simulink model "PCC_NoGearOpt_Revision"  (R2020a)
settings: Solver=ode45  StartTime=0.0  StopTime=3000  RelTol=1e-3
PreLoadFcn:
  | initial
PostLoadFcn:
  | initial
InitFcn:
  | initial
model workspace (MAT data in the model file):
  Af = Simulink.Signal
  Af.DataType = 'double'
  Af.Dimensions = -1
  Af.DimensionsMode = 'auto'
  Af.Complexity = 'real'
  Af.SampleTime = -1
  Af.SamplingMode = 'auto'
  Af.InitialValue = '4.2'
  CD = Simulink.Signal
  CD.DataType = 'double'
  CD.Dimensions = -1
  CD.DimensionsMode = 'auto'
  CD.Complexity = 'real'
  CD.SampleTime = -1
  CD.SamplingMode = 'auto'
  CD.InitialValue = '0.5'
  Delta_t = Simulink.Signal
  Delta_t.DataType = 'double'
  Delta_t.Dimensions = -1
  Delta_t.DimensionsMode = 'auto'
  Delta_t.Complexity = 'real'
  Delta_t.SampleTime = -1
  Delta_t.SamplingMode = 'auto'
  Delta_t.InitialValue = '1'
  If = Simulink.Signal
  If.DataType = 'double'
  If.Dimensions = -1
  If.DimensionsMode = 'auto'
  If.Complexity = 'real'
  If.SampleTime = -1
  If.SamplingMode = 'auto'
  If.InitialValue = '2.87'
  Ig = Simulink.Signal
  Ig.DataType = 'double'
  Ig.Dimensions = 14
  Ig.DimensionsMode = 'auto'
  Ig.Complexity = 'real'
  Ig.SampleTime = -1
  Ig.SamplingMode = 'auto'
  Ig.InitialValue = '[16.41,13.16,11.13,8.92,7.16,5.74,4.68,3.75,2.97,2.38,1.91,1.53,1.25,1]'
  L00 = Simulink.Signal
  L00.DataType = 'double'
  L00.Dimensions = -1
  L00.DimensionsMode = 'auto'
  L00.Complexity = 'real'
  L00.SampleTime = -1
  L00.SamplingMode = 'auto'
  L00.InitialValue = '-1.522'
  L01 = Simulink.Signal
  L01.DataType = 'double'
  L01.Dimensions = -1
  L01.DimensionsMode = 'auto'
  L01.Complexity = 'real'
  L01.SampleTime = -1
  L01.SamplingMode = 'auto'
  L01.InitialValue = '0.002239'
  L02 = Simulink.Signal
  L02.DataType = 'double'
  L02.Dimensions = -1
  L02.DimensionsMode = 'auto'
  L02.Complexity = 'real'
  L02.SampleTime = -1
  L02.SamplingMode = 'auto'
  L02.InitialValue = '-2.185e-07'
  L10 = Simulink.Signal
  L10.DataType = 'double'
  L10.Dimensions = -1
  L10.DimensionsMode = 'auto'
  L10.Complexity = 'real'
  L10.SampleTime = -1
  L10.SamplingMode = 'auto'
  L10.InitialValue = '0.002321'
  L11 = Simulink.Signal
  L11.DataType = 'double'
  L11.Dimensions = -1
  L11.DimensionsMode = 'auto'
  L11.Complexity = 'real'
  L11.SampleTime = -1
  L11.SamplingMode = 'auto'
  L11.InitialValue = '1.94e-06'
  L12 = Simulink.Signal
  L12.DataType = 'double'
  L12.Dimensions = -1
  L12.DimensionsMode = 'auto'
  L12.Complexity = 'real'
  L12.SampleTime = -1
  L12.SamplingMode = 'auto'
  L12.InitialValue = '4.879e-10'
  L20 = Simulink.Signal
  L20.DataType = 'double'
  L20.Dimensions = -1
  L20.DimensionsMode = 'auto'
  L20.Complexity = 'real'
  L20.SampleTime = -1
  L20.SamplingMode = 'auto'
  L20.InitialValue = '7.602e-07'
  L21 = Simulink.Signal
  L21.DataType = 'double'
  L21.Dimensions = -1
  L21.DimensionsMode = 'auto'
  L21.Complexity = 'real'
  L21.SampleTime = -1
  L21.SamplingMode = 'auto'
  L21.InitialValue = '-1.465e-09'
  L22 = Simulink.Signal
  L22.DataType = 'double'
  L22.Dimensions = -1
  L22.DimensionsMode = 'auto'
  L22.Complexity = 'real'
  L22.SampleTime = -1
  L22.SamplingMode = 'auto'
  L22.InitialValue = '9.135e-13'
  M = Simulink.Signal
  M.DataType = 'double'
  M.Dimensions = -1
  M.DimensionsMode = 'auto'
  M.Complexity = 'real'
  M.SampleTime = -1
  M.SamplingMode = 'auto'
  M.InitialValue = '49000'
  Np = Simulink.Signal
  Np.DataType = 'double'
  Np.Dimensions = -1
  Np.DimensionsMode = 'auto'
  Np.Complexity = 'real'
  Np.SampleTime = -1
  Np.SamplingMode = 'auto'
  Np.InitialValue = '50'
  Tb_min = Simulink.Signal
  Tb_min.DataType = 'double'
  Tb_min.Dimensions = -1
  Tb_min.DimensionsMode = 'auto'
  Tb_min.Complexity = 'real'
  Tb_min.SampleTime = -1
  Tb_min.SamplingMode = 'auto'
  Tb_min.InitialValue = '-20000'
  Te_max = Simulink.Signal
  Te_max.DataType = 'double'
  Te_max.Dimensions = -1
  Te_max.DimensionsMode = 'auto'
  Te_max.Complexity = 'real'
  Te_max.SampleTime = -1
  Te_max.SamplingMode = 'auto'
  Te_max.InitialValue = '2650'
  Te_min = Simulink.Signal
  Te_min.DataType = 'double'
  Te_min.Dimensions = -1
  Te_min.DimensionsMode = 'auto'
  Te_min.Complexity = 'real'
  Te_min.SampleTime = -1
  Te_min.SamplingMode = 'auto'
  Te_min.InitialValue = '-400'
  eta = Simulink.Signal
  eta.DataType = 'double'
  eta.Dimensions = -1
  eta.DimensionsMode = 'auto'
  eta.Complexity = 'real'
  eta.SampleTime = -1
  eta.SamplingMode = 'auto'
  eta.InitialValue = '0.98'
  f = Simulink.Signal
  f.DataType = 'double'
  f.Dimensions = -1
  f.DimensionsMode = 'auto'
  f.Complexity = 'real'
  f.SampleTime = -1
  f.SamplingMode = 'auto'
  f.InitialValue = '0.00743'
  g = Simulink.Signal
  g.DataType = 'double'
  g.Dimensions = -1
  g.DimensionsMode = 'auto'
  g.Complexity = 'real'
  g.SampleTime = -1
  g.SamplingMode = 'auto'
  g.InitialValue = '9.8'
  kappa_1 = Simulink.Signal
  kappa_1.DataType = 'double'
  kappa_1.Dimensions = -1
  kappa_1.DimensionsMode = 'auto'
  kappa_1.Complexity = 'real'
  kappa_1.SampleTime = -1
  kappa_1.SamplingMode = 'auto'
  kappa_1.InitialValue = '1'
  kappa_2 = Simulink.Signal
  kappa_2.DataType = 'double'
  kappa_2.Dimensions = -1
  kappa_2.DimensionsMode = 'auto'
  kappa_2.Complexity = 'real'
  kappa_2.SampleTime = -1
  kappa_2.SamplingMode = 'auto'
  kappa_2.InitialValue = '0.05'
  rho = Simulink.Signal
  rho.DataType = 'double'
  rho.Dimensions = -1
  rho.DimensionsMode = 'auto'
  rho.Complexity = 'real'
  rho.SampleTime = -1
  rho.SamplingMode = 'auto'
  rho.InitialValue = '1.225'
  rw = Simulink.Signal
  rw.DataType = 'double'
  rw.Dimensions = -1
  rw.DimensionsMode = 'auto'
  rw.Complexity = 'real'
  rw.SampleTime = -1
  rw.SamplingMode = 'auto'
  rw.InitialValue = '0.5267'
values from neighbouring files (symbols this model uses):
  EngMinTrq_Para_Value = -400    [initial.m]
  GearIni_Para_Value = 12    [initial.m]
  ParaMAP_RdSlopeOffsetAll = RdSlopeOffsetAll(5,1:2094)    [initial.m]
  ParaMAP_RdSlopeValueAll = RdSlopeValueAll(5,1:2094)    [initial.m]
  Rd_LeaderSpd = [19.4444444444 19.7511370506 20.5925623188 20.8767591057 20.2737444786 20.4902746731 20.4442142988 20.3221868298 20.2125924983 19.7727091401 19.6123069776 19.2200993307 ... (126 elements, 126x1)]    [RdLeaderSpdData.mat]
  Rd_Pos = [0:20:2500]    [LeaderSpd_Generate.m]    (also in RdLeaderSpdData.mat = [0 20 40 60 80 100 120 140 160 180 200 220 ... (126 elements)
undefined symbols (not defined in the file or in its folder): sigbuilder_block
libraries: simulink x4, Solver_SF x1
(part 1 of 2)
settings Model: SimulationMode=accelerator  Creator=LH  LastModifiedBy=luoro
settings DataIOCC: LimitDataPoints=on  SaveFormat=Array  ReturnWorkspaceOutputsName=PCC
settings OptimizationCC: BlockReduction=off  BooleanDataType=off  LifeSpan=inf
settings DebuggingCC: SaveWithParameterizedLinksMsg=none  UnderspecifiedInitializationDetection=Classic  MergeDetectMultiDrivingBlocksExec=none  SignalResolutionControl=TryResolveAllWithWarning  SFUnexpectedBacktrackingDiag=warning  SFNoUnconditionalDefaultTransitionDiag=warning  SFExecutionAtInitializationDiag=none  ArithmeticOperatorsInVariantConditions=warning
settings HardwareCC: ProdBitPerPointer=32  ProdBitPerSizeT=32  ProdBitPerPtrDiffT=32  ProdLargestAtomicFloat=None  ProdIntDivRoundTo=Undefined  ProdEndianess=Unspecified  ProdWordSize=32  ProdHWDeviceType=32-bit Generic  TargetBitPerPointer=64  TargetBitPerSizeT=64  TargetBitPerPtrDiffT=64  TargetLongLongMode=on  TargetIntDivRoundTo=Zero  TargetEndianess=LittleEndian  TargetWordSize=64  TargetHWDeviceType=MATLAB Host  ProdEqTarget=off
settings ModelReferenceCC: PropagateSignalLabelsOutOfModel=off
settings SFSimCC: SimUseLocalCustomCode=off  CustomCodeUndefinedFunction=UseInterfaceOnly
settings RTWCC: RTWUseLocalCustomCode=off
settings CodeAppCC: StateflowObjectComments=on
settings GRTTargetCC: TargetLangStandard=C89/C90 (ANSI)
settings ConfigComp: CovMetricSettings=dw  CovSaveCumulativeToWorkspaceVar=on  CovSaveSingleToWorkspaceVar=on  CovExternalEMLEnable=off  CovSFcnEnable=off

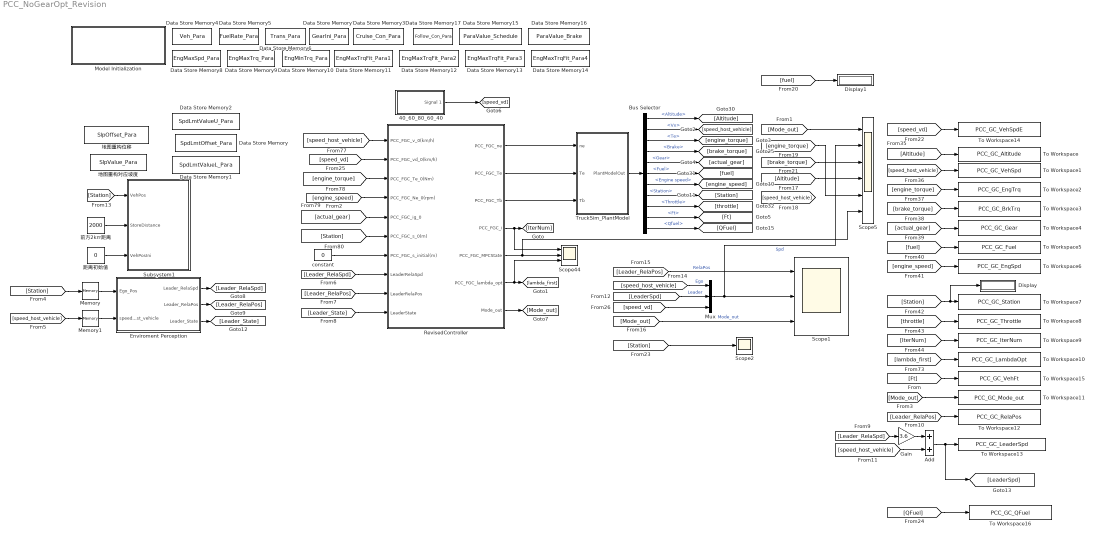
== system PCC_NoGearOpt_Revision ==
  40_60_80_60_40 : Subsystem  Tag=STV Subsys  LoadFcn=sigbuilder_block('load');  StartFcn=sigbuilder_block('start');  StopFcn=sigbuilder_block('stop');  ClipboardFcn=sigbuilder_block('clipboard');  mask(Sigbuilder block){tuvar=[0:10]}
      mask help: Simulink:masks:SigbuilderBlock_MD
      mask init:
      | if ~strcmp(get_param(bdroot(gcbh),'SimulationStatus'),'stopped') tuvar = sigbuilder_block('maskInit'); end
      settings: CopyFcn=sigbuilder_block('copy');  DeleteFcn=sigbuilder_block('delete');  ModelCloseFcn=sigbuilder_block('modelClose');  PreSaveFcn=sigbuilder_block('preSave');  PauseFcn=sigbuilder_block('pause');  ContinueFcn=sigbuilder_block('continue');  NameChangeFcn=sigbuilder_block('namechange');  OpenFcn=sigbuilder_block('open',[0 30 1440 721.5 ]);  CloseFcn=sigbuilder_block('close');
      mask Display: plot(0, 0, 100, 100,[2, 2, 32, 32, 2], [68, 8, 8, 68, 68],[32, 2], [38, 38], [32, 19, 2],[53, 60, 44], [32, 17, 17, 2],[16, 16, 31, 31]);txt = getActiveGroup(gcbh);text(2, 100, txt,'verticalAlignment', 'top');
  Add : Sum
  Bus Selector : BusSelector  OutputSignals=Altitude,Vx,Te,Brake,Gear,Fuel,Engine speed,Station,Throttle,Ft,Qfuel
  Data Store Memory : DataStoreMemory  DataStoreName=SpdLmtOffset_Para  InitialValue=ParaMAP_RdSpdLimitOffset  ShowAdditionalParam=off  OutDataTypeStr=double
  Data Store Memory1 : DataStoreMemory  DataStoreName=SpdLmtValueL_Para  InitialValue=ParaMAP_RdSpdLimitL  ShowAdditionalParam=off  OutDataTypeStr=double
  Data Store Memory10 : DataStoreMemory  DataStoreName=EngMinTrq_Para  ReadBeforeWriteMsg=warning  WriteAfterWriteMsg=warning  WriteAfterReadMsg=warning  InitialValue=EngMinTrq_Para_Value  ShowAdditionalParam=off  OutDataTypeStr=double
  Data Store Memory11 : DataStoreMemory  DataStoreName=EngMaxTrqFit_Para1  ReadBeforeWriteMsg=warning  WriteAfterWriteMsg=warning  WriteAfterReadMsg=warning  InitialValue=EngMaxTrqFit_Para_Value1  ShowAdditionalParam=off  OutDataTypeStr=double
  Data Store Memory12 : DataStoreMemory  DataStoreName=EngMaxTrqFit_Para2  ReadBeforeWriteMsg=warning  WriteAfterWriteMsg=warning  WriteAfterReadMsg=warning  InitialValue=EngMaxTrqFit_Para_Value2  ShowAdditionalParam=off  OutDataTypeStr=double
  Data Store Memory13 : DataStoreMemory  DataStoreName=EngMaxTrqFit_Para3  ReadBeforeWriteMsg=warning  WriteAfterWriteMsg=warning  WriteAfterReadMsg=warning  InitialValue=EngMaxTrqFit_Para_Value3  ShowAdditionalParam=off  OutDataTypeStr=double
  Data Store Memory14 : DataStoreMemory  DataStoreName=EngMaxTrqFit_Para4  ReadBeforeWriteMsg=warning  WriteAfterWriteMsg=warning  WriteAfterReadMsg=warning  InitialValue=EngMaxTrqFit_Para_Value4  ShowAdditionalParam=off  OutDataTypeStr=double
  Data Store Memory15 : DataStoreMemory  DataStoreName=ParaValue_Schedule  ReadBeforeWriteMsg=warning  WriteAfterWriteMsg=warning  WriteAfterReadMsg=warning  InitialValue=ParaValue_Schedule  ShowAdditionalParam=off  OutDataTypeStr=double
  Data Store Memory16 : DataStoreMemory  DataStoreName=ParaValue_Brake  ReadBeforeWriteMsg=warning  WriteAfterWriteMsg=warning  WriteAfterReadMsg=warning  InitialValue=ParaValue_Brake  ShowAdditionalParam=off  OutDataTypeStr=double
  Data Store Memory17 : DataStoreMemory  DataStoreName=Follow_Con_Para  ReadBeforeWriteMsg=warning  WriteAfterWriteMsg=warning  WriteAfterReadMsg=warning  InitialValue=Follow_Con_Para_Value  ShowAdditionalParam=off  OutDataTypeStr=double
  Data Store Memory2 : DataStoreMemory  DataStoreName=SpdLmtValueU_Para  InitialValue=ParaMAP_RdSpdLimitU  ShowAdditionalParam=off  OutDataTypeStr=double
  Data Store Memory3 : DataStoreMemory  DataStoreName=Cruise_Con_Para  ReadBeforeWriteMsg=warning  WriteAfterWriteMsg=warning  WriteAfterReadMsg=warning  InitialValue=Cruise_Con_Para_Value  ShowAdditionalParam=off  OutDataTypeStr=double
  Data Store Memory4 : DataStoreMemory  DataStoreName=Veh_Para  ReadBeforeWriteMsg=warning  WriteAfterWriteMsg=warning  WriteAfterReadMsg=warning  InitialValue=Veh_Para_Value  ShowAdditionalParam=off  OutDataTypeStr=double
  Data Store Memory5 : DataStoreMemory  DataStoreName=FuelRate_Para  ReadBeforeWriteMsg=warning  WriteAfterWriteMsg=warning  WriteAfterReadMsg=warning  InitialValue=FuelRate_Para_Value  ShowAdditionalParam=off  OutDataTypeStr=double
  Data Store Memory6 : DataStoreMemory  DataStoreName=Trans_Para  ReadBeforeWriteMsg=warning  WriteAfterWriteMsg=warning  WriteAfterReadMsg=warning  InitialValue=Trans_Para_Value  ShowAdditionalParam=off  OutDataTypeStr=double
  Data Store Memory7 : DataStoreMemory  DataStoreName=GearIni_Para  ReadBeforeWriteMsg=warning  WriteAfterWriteMsg=warning  WriteAfterReadMsg=warning  InitialValue=GearIni_Para_Value  ShowAdditionalParam=off  OutDataTypeStr=double
  Data Store Memory8 : DataStoreMemory  DataStoreName=EngMaxSpd_Para  ReadBeforeWriteMsg=warning  WriteAfterWriteMsg=warning  WriteAfterReadMsg=warning  InitialValue=EngMaxSpd_Para_Value  ShowAdditionalParam=off  OutDataTypeStr=double
  Data Store Memory9 : DataStoreMemory  DataStoreName=EngMaxTrq_Para  ReadBeforeWriteMsg=warning  WriteAfterWriteMsg=warning  WriteAfterReadMsg=warning  InitialValue=EngMaxTrq_Para_Value  ShowAdditionalParam=off  OutDataTypeStr=double
  Display : Display
      settings: Format=bank
  Display1 : Display
      settings: Format=bank
  Enviroment Perception : Subsystem
  Gain : Gain  Gain=3.6
  Memory : Memory
  Memory1 : Memory  InitialCondition=60
  Model Initialization : Subsystem  AncestorBlock=artemis/Tools /Misc/Model Initialization  mask(Model Functions){InitFcnX=initial, prel=on, posl=on, inif=on, strf=off}
      mask prompts: InitFcnX "Initialisation"; prel "Preload Function"; posl "PostLoad Function"; inif "InitFcn"; strf "StartFcn"
      mask init:
      | currentBlock = gcb;
      | root = bdroot(currentBlock);
      | 
      | if ~strcmp(get_param(root,'BlockDiagramType'),'library')
      |     if prel==1
      |         set_param(root, 'PreLoadFcn', InitFcnX);
      |     else
      |         set_param(root, 'PreLoadFcn', '');
      |     end
      |     if inif==1
      |         set_param(root, 'InitFcn', InitFcnX);
      |     else
      |         set_param(root, 'InitFcn', '');
      |     end
      |     if strf==1
      |         set_param(root, 'StartFcn', InitFcnX);
      |     else
      |         set_param(root, 'StartFcn', '');
      |     end
      |     if posl==1
      |         set_param(root, 'PostLoadFcn', InitFcnX);
      |     else
      |         set_param(root, 'PostLoadFcn', '');
      |     end
      | end
      | 
      | pos = get_param(currentBlock, 'Position');
      | width = pos(3) - pos(1); height = pos(4) - pos(2);
      | txt = [ upper(root) '\n' '- InitFcn. . . . . '  get_param(root, 'InitFcn') ];
      settings: CopyFcn=set_param(gcb,'LinkStatus','inactive')
      mask Display: text(5, height*0.5, txt, 'horizontalAlignment', 'left', 'verticalAlignment', 'middle') ;
  Mux : Mux  Inputs=3
  RevisedController : Subsystem
  Scope1 : Scope  NumInputPorts=3
  Scope2 : Scope
  Scope44 : Scope  NumInputPorts=3
  Scope5 : Scope  NumInputPorts=6
  Subsystem1 : Subsystem
  To Workspace : ToWorkspace  VariableName=PCC_GC_Altitude  SaveFormat=Structure With Time  SampleTime=0.01
      settings: Save2DSignal=2-D array (concatenate along first dimension)
  To Workspace1 : ToWorkspace  VariableName=PCC_GC_VehSpd  SaveFormat=Structure With Time  SampleTime=0.01
  To Workspace10 : ToWorkspace  VariableName=PCC_GC_LambdaOpt  SaveFormat=Structure With Time  SampleTime=0.01
  To Workspace11 : ToWorkspace  VariableName=PCC_GC_Mode_out  SaveFormat=Structure With Time  SampleTime=0.01
  To Workspace12 : ToWorkspace  VariableName=PCC_GC_RelaPos  SaveFormat=Structure With Time  SampleTime=0.01
  To Workspace13 : ToWorkspace  VariableName=PCC_GC_LeaderSpd  SaveFormat=Structure With Time  SampleTime=0.01
  To Workspace14 : ToWorkspace  VariableName=PCC_GC_VehSpdE  SaveFormat=Structure With Time  SampleTime=0.01
  To Workspace15 : ToWorkspace  VariableName=PCC_GC_VehFt  SaveFormat=Structure With Time  SampleTime=0.01
  To Workspace16 : ToWorkspace  VariableName=PCC_GC_QFuel  SaveFormat=Structure With Time  SampleTime=0.01
  To Workspace2 : ToWorkspace  VariableName=PCC_GC_EngTrq  SaveFormat=Structure With Time  SampleTime=0.01
  To Workspace3 : ToWorkspace  VariableName=PCC_GC_BrkTrq  SaveFormat=Structure With Time  SampleTime=0.01
  To Workspace4 : ToWorkspace  VariableName=PCC_GC_Gear  SaveFormat=Structure With Time  SampleTime=0.01
  To Workspace5 : ToWorkspace  VariableName=PCC_GC_Fuel  SaveFormat=Structure With Time  SampleTime=0.01
  To Workspace6 : ToWorkspace  VariableName=PCC_GC_EngSpd  SaveFormat=Structure With Time  SampleTime=0.01
  To Workspace7 : ToWorkspace  VariableName=PCC_GC_Station  SaveFormat=Structure With Time  SampleTime=0.01
  To Workspace8 : ToWorkspace  VariableName=PCC_GC_Throttle  SaveFormat=Structure With Time  SampleTime=0.01
  To Workspace9 : ToWorkspace  VariableName=PCC_GC_IterNum  SaveFormat=Structure With Time  SampleTime=0.01
  TruckSim_PlantModel : Subsystem
  constant : Constant  Value=0
  前方2km距离 : Constant  Value=2000
  地图重构位移 : DataStoreMemory  DataStoreName=SlpOffset_Para  InitialValue=ParaMAP_RdSlopeOffsetFirst200  ShowAdditionalParam=off  OutDataTypeStr=double
  地图重构对应坡度 : DataStoreMemory  DataStoreName=SlpValue_Para  InitialValue=ParaMAP_RdSlopeValueFirst200  ShowAdditionalParam=off  OutDataTypeStr=double
  距离初始值 : Constant  Value=0
  wires:
  [Altitude] -> Scope5/4
  [engine_torque] -> Scope5/5
  [fuel] -> Display1/1
  [Altitude] -> To Workspace/1
  [speed_host_vehicle] -> To Workspace1/1
  [engine_torque] -> To Workspace2/1
  [brake_torque] -> To Workspace3/1
  [actual_gear] -> To Workspace4/1
  [fuel] -> To Workspace5/1
  [engine_speed] -> To Workspace6/1
  [Station] -> Display/1, To Workspace7/1
  [throttle] -> To Workspace8/1
  [IterNum] -> To Workspace9/1
  [Station] -> Subsystem1/1(VehPos)
  前方2km距离/1 -> Subsystem1/2(StoreDistance)
  距离初始值/1 -> Subsystem1/3(VehPosIni)
  [lambda_first] -> To Workspace10/1
  RevisedController/1(PCC_FGC_ne) -> TruckSim_PlantModel/1(ne)
  RevisedController/2(PCC_FGC_Te) -> TruckSim_PlantModel/2(Te)
  [speed_host_vehicle] -> RevisedController/1(PCC_FGC_v_0(km/h))
  [engine_torque] -> RevisedController/3(PCC_FGC_Te_0(Nm))
  [actual_gear] -> RevisedController/5(PCC_FGC_ig_0)
  [Station] -> RevisedController/6(PCC_FGC_s_0(m))
  constant/1 -> RevisedController/7(PCC_FGC_s_initial(m))
  TruckSim_PlantModel/1(PlantModelOut) -> Bus Selector/1
  Bus Selector/2 -> [speed_host_vehicle]  "<Vx>"
  Bus Selector/1 -> [Altitude]  "<Altitude>"
  Bus Selector/3 -> [engine_torque]  "<Te>"
  Bus Selector/4 -> [brake_torque]  "<Brake>"
  Bus Selector/5 -> [actual_gear]  "<Gear>"
  Bus Selector/6 -> [fuel]  "<Fuel>"
  Bus Selector/7 -> [engine_speed]  "<Engine speed>"
  Bus Selector/8 -> [Station]  "<Station>"
  Bus Selector/9 -> [throttle]  "<Throttle>"
  Bus Selector/10 -> [Ft]  "<Ft>"
  [Ft] -> To Workspace15/1
  [Mode_out] -> Scope5/1
  RevisedController/4(PCC_FGC_i) -> [IterNum], Scope44/1
  RevisedController/5(PCC_FGC_MPCState) -> Scope5/6, Scope44/2
  RevisedController/6(PCC_FGC_lambda_opt) -> Scope44/3, [lambda_first]
  [engine_speed] -> RevisedController/4(PCC_FGC_Ne_0(rpm))
  RevisedController/3(PCC_FGC_Tb) -> TruckSim_PlantModel/3(Tb)
  RevisedController/7(Mode_out) -> [Mode_out]
  [Mode_out] -> To Workspace11/1
  [Leader_RelaSpd] -> RevisedController/8(LeaderRelaSpd)
  [Leader_RelaPos] -> RevisedController/9(LeaderRelaPos)
  [Leader_State] -> RevisedController/10(LeaderState)
  [speed_host_vehicle] -> Memory1/1
  [Station] -> Memory/1
  Enviroment Perception/1(Leader_RelaSpd) -> [Leader_RelaSpd]
  Enviroment Perception/2(Leader_RelaPos) -> [Leader_RelaPos]
  Enviroment Perception/3(Leader_State) -> [Leader_State]
  [Leader_RelaSpd] -> Gain/1
  Add/1 -> [LeaderSpd], To Workspace13/1
  Gain/1 -> Add/1
  [Leader_RelaPos] -> To Workspace12/1
  [speed_host_vehicle] -> Add/2
  [LeaderSpd] -> Mux/2  "Leader"
  Mux/1 -> Scope5/2, Scope1/2  "Spd"
  [speed_host_vehicle] -> Mux/1  "Ego"
  [Leader_RelaPos] -> Scope1/1  "RelaPos"
  [Mode_out] -> Scope1/3  "Mode_out"
  Memory/1 -> Enviroment Perception/1(Ego_Pos)
  Memory1/1 -> Enviroment Perception/2(speed_host_vehicle)
  [speed_vd] -> To Workspace14/1
  [Station] -> Scope2/1
  Bus Selector/11 -> [QFuel]  "<Qfuel>"
  [QFuel] -> To Workspace16/1
  [speed_vd] -> RevisedController/2(PCC_FGC_vd_0(km/h))
  [speed_vd] -> Mux/3
  40_60_80_60_40/1(Signal 1) -> [speed_vd]
  [brake_torque] -> Scope5/3

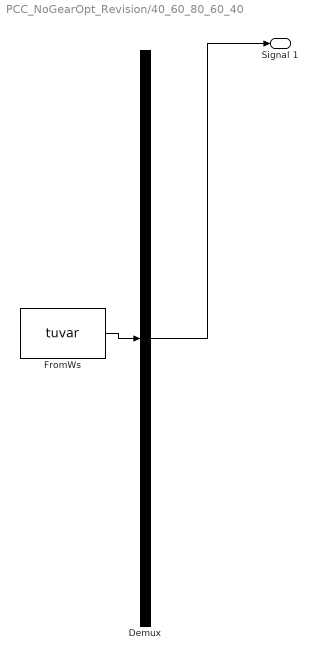
== system PCC_NoGearOpt_Revision/40_60_80_60_40 ==
  Demux : Demux  Tag=STV Demux  Outputs=1
      settings: DisplayOption=none
  FromWs : FromWorkspace  Tag=STV FromWs  VariableName=tuvar
      SigBuilderData=|
      | common.afterFinalStr = 'Extrapolate'
      | common.sampleTime = 0
      | dataSet.timeRange = [0 2000]
      | dataSet.name = 'Group 1'
      | sbobj.Groups.Name = 'Group 1'
      | sbobj.Groups.Signals.Name = 'Signal 1'
      | sbobj.Groups.Signals.XData = [0 300 300 1200 1600 2000]
      | sbobj.Groups.Signals.YData = [80 80 80 80 80 80]
      | sbobj.Groups.TimeRange = [0 2000]
  Signal 1 : Outport  Tag=STV Outport
  wires:
  Demux/1 -> Signal 1/1
  FromWs/1 -> Demux/1

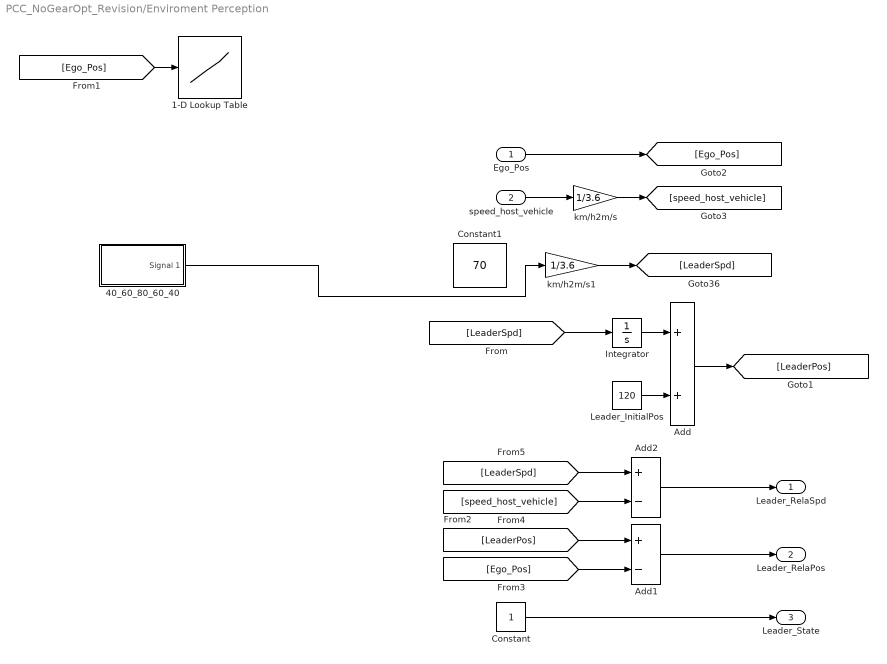
== system PCC_NoGearOpt_Revision/Enviroment Perception ==
  Ego_Pos : Inport
  speed_host_vehicle : Inport  Port=2
  1-D Lookup Table : Lookup_n-D  NumberOfTableDimensions=1  BreakpointsForDimension1=Rd_Pos  Table=Rd_LeaderSpd  InternalRulePriority=Speed  RndMeth=Simplest  InputSameDT=on
  40_60_80_60_40 : Subsystem  Tag=STV Subsys  LoadFcn=sigbuilder_block('load');  StartFcn=sigbuilder_block('start');  StopFcn=sigbuilder_block('stop');  ClipboardFcn=sigbuilder_block('clipboard');  mask(Sigbuilder block){tuvar=[0:10]}
      mask help: Simulink:masks:SigbuilderBlock_MD
      mask init:
      | if ~strcmp(get_param(bdroot(gcbh),'SimulationStatus'),'stopped') tuvar = sigbuilder_block('maskInit'); end
      settings: CopyFcn=sigbuilder_block('copy');  DeleteFcn=sigbuilder_block('delete');  ModelCloseFcn=sigbuilder_block('modelClose');  PreSaveFcn=sigbuilder_block('preSave');  PauseFcn=sigbuilder_block('pause');  ContinueFcn=sigbuilder_block('continue');  NameChangeFcn=sigbuilder_block('namechange');  OpenFcn=sigbuilder_block('open',[6 30 1428 680.25 ]);  CloseFcn=sigbuilder_block('close');
      mask Display: plot(0, 0, 100, 100,[2, 2, 32, 32, 2], [68, 8, 8, 68, 68],[32, 2], [38, 38], [32, 19, 2],[53, 60, 44], [32, 17, 17, 2],[16, 16, 31, 31]);txt = getActiveGroup(gcbh);text(2, 100, txt,'verticalAlignment', 'top');
  Add : Sum
  Add1 : Sum  Inputs=+-
  Add2 : Sum  Inputs=+-
  Constant : Constant
  Constant1 : Constant  Value=70
  Integrator : Integrator
  Leader_InitialPos : Constant  Value=120
  km/h2m/s : Gain  Gain=1/3.6
  km/h2m/s1 : Gain  Gain=1/3.6
  Leader_RelaSpd : Outport
  Leader_RelaPos : Outport  Port=2
  Leader_State : Outport  Port=3
  wires:
  Ego_Pos/1 -> [Ego_Pos]
  [LeaderSpd] -> Integrator/1
  Integrator/1 -> Add/1
  Add/1 -> [LeaderPos]
  Leader_InitialPos/1 -> Add/2
  [LeaderPos] -> Add1/1
  [Ego_Pos] -> Add1/2
  speed_host_vehicle/1 -> km/h2m/s/1
  Add1/1 -> Leader_RelaPos/1
  km/h2m/s/1 -> [speed_host_vehicle]
  [LeaderSpd] -> Add2/1
  Add2/1 -> Leader_RelaSpd/1
  [speed_host_vehicle] -> Add2/2
  Constant/1 -> Leader_State/1
  [Ego_Pos] -> 1-D Lookup Table/1
  km/h2m/s1/1 -> [LeaderSpd]
  40_60_80_60_40/1(Signal 1) -> km/h2m/s1/1

== system PCC_NoGearOpt_Revision/Model Initialization ==

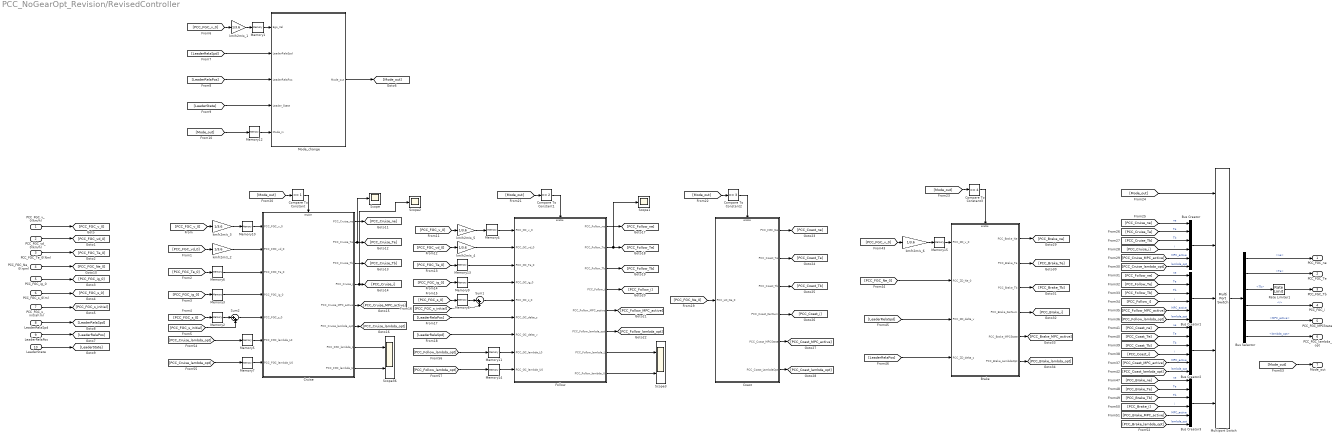
== system PCC_NoGearOpt_Revision/RevisedController ==
  PCC_FGC_v_0(km/h) : Inport
  PCC_FGC_vd_0(km/h) : Inport  Port=2
  PCC_FGC_Te_0(Nm) : Inport  Port=3
  PCC_FGC_Ne_0(rpm) : Inport  Port=4
  PCC_FGC_ig_0 : Inport  Port=5
  PCC_FGC_s_0(m) : Inport  Port=6
  PCC_FGC_s_initial(m) : Inport  Port=7
  LeaderRelaSpd : Inport  Port=8
  LeaderRelaPos : Inport  Port=9
  LeaderState : Inport  Port=10
  Brake : Subsystem
  Bus Creator{,1..3} (4 alike) : BusCreator  Inputs=6
  Bus Selector : BusSelector  OutputSignals=ne,Te,Tb,i,MPC_active,lambda_opt
  Coast : Subsystem  TreatAsAtomicUnit=on
  Compare To Constant : simulink/Logic and Bit Operations/Compare To Constant  relop===  const=1  OutDataTypeStr=boolean
  Compare To Constant1 : simulink/Logic and Bit Operations/Compare To Constant  relop===  const=2  OutDataTypeStr=boolean
  Compare To Constant2 : simulink/Logic and Bit Operations/Compare To Constant  relop===  const=3  OutDataTypeStr=boolean
  Compare To Constant3 : simulink/Logic and Bit Operations/Compare To Constant  relop===  const=4  OutDataTypeStr=boolean
  Cruise : Subsystem
  Follow : Subsystem
  Memory{1,4,10,15} (4 alike) : Memory  InitialCondition=60/3.6
  Memory11 : Memory  InitialCondition=-5000
  Memory12 : Memory  InitialCondition=1
  Memory{2,6,8,13} (4 alike) : Memory
  Memory14 : Memory  InitialCondition=5000
  Memory3 : Memory  InitialCondition=12
  Memory5 : Memory  InitialCondition=-5000
  Memory7 : Memory  InitialCondition=5000
  Memory9 : Memory  InitialCondition=12
  Mode_change : MATLAB Function  TreatAsAtomicUnit=on
  Multiport Switch : MultiPortSwitch  Inputs=4
  Rate Limiter1 : RateLimiter  RisingSlewLimit=700  FallingSlewLimit=-700  SampleTimeMode=inherited
  Scope : Scope
  Scope1 : Scope
  Scope2 : Scope
  Scope3 : Scope  NumInputPorts=2
  Scope36 : Scope  NumInputPorts=2
  Sum1 : Sum  Inputs=|++
  Sum2 : Sum  Inputs=|++
  km/h2m/s_{1..6} (6 alike) : Gain  Gain=1/3.6
  PCC_FGC_ne : Outport  VectorParamsAs1DForOutWhenUnconnected=off
  PCC_FGC_Te : Outport  Port=2  VectorParamsAs1DForOutWhenUnconnected=off
  PCC_FGC_Tb : Outport  Port=3  VectorParamsAs1DForOutWhenUnconnected=off
  PCC_FGC_i : Outport  Port=4  VectorParamsAs1DForOutWhenUnconnected=off
  PCC_FGC_MPCState : Outport  Port=5  VectorParamsAs1DForOutWhenUnconnected=off
  PCC_FGC_lambda_opt : Outport  Port=6  VectorParamsAs1DForOutWhenUnconnected=off
  Mode_out : Outport  Port=7
  wires:
  km/h2m/s_3/1 -> Memory10/1
  PCC_FGC_vd_0(km/h)/1 -> [PCC_FGC_vd_0]
  Memory2/1 -> Sum2/1
  PCC_FGC_s_initial(m)/1 -> [PCC_FGC_s_initial]
  PCC_FGC_Te_0(Nm)/1 -> [PCC_FGC_Te_0]
  PCC_FGC_v_0(km/h)/1 -> [PCC_FGC_v_0]
  PCC_FGC_ig_0/1 -> [PCC_FGC_ig_0]
  PCC_FGC_s_0(m)/1 -> [PCC_FGC_s_0]
  [PCC_FGC_v_0] -> km/h2m/s_3/1
  [PCC_FGC_vd_0] -> km/h2m/s_2/1
  [PCC_FGC_Te_0] -> Memory6/1
  [PCC_FGC_ig_0] -> Memory3/1
  [PCC_FGC_s_0] -> Memory2/1
  [PCC_FGC_s_initial] -> Sum2/2
  Bus Selector/1 -> PCC_FGC_ne/1  "<ne>"
  Bus Selector/2 -> PCC_FGC_Te/1  "<Te>"
  Bus Selector/6 -> PCC_FGC_lambda_opt/1  "<lambda_opt>"
  Bus Selector/5 -> PCC_FGC_MPCState/1  "<MPC_active>"
  Bus Selector/4 -> PCC_FGC_i/1  "<i>"
  LeaderRelaSpd/1 -> [LeaderRelaSpd]
  LeaderRelaPos/1 -> [LeaderRelaPos]
  LeaderState/1 -> [LeaderState]
  [PCC_FGC_v_0] -> km/h2m/s_1/1
  km/h2m/s_1/1 -> Memory1/1
  Memory1/1 -> Mode_change/1(Ego_Vel)
  [LeaderRelaSpd] -> Mode_change/2(LeaderRelaSpd)
  [LeaderRelaPos] -> Mode_change/3(LeaderRelaPos)
  [LeaderState] -> Mode_change/4(Leader_State)
  Mode_change/1(Mode_out) -> [Mode_out]
  Memory12/1 -> Mode_change/5(Mode_in)
  [Mode_out] -> Memory12/1
  [PCC_FGC_ig_0] -> Memory9/1
  [PCC_FGC_v_0] -> km/h2m/s_5/1
  Memory8/1 -> Sum1/1
  [PCC_FGC_s_initial] -> Sum1/2
  [PCC_FGC_s_0] -> Memory8/1
  km/h2m/s_5/1 -> Memory4/1
  [PCC_FGC_vd_0] -> km/h2m/s_4/1
  [PCC_FGC_Te_0] -> Memory13/1
  Cruise/7(PCC_FGC_lambda_L) -> Scope36/1
  Cruise/8(PCC_FGC_lambda_U) -> Scope36/2
  Memory10/1 -> Cruise/1(PCC_FGC_v_0)
  km/h2m/s_2/1 -> Cruise/2(PCC_FGC_vd_0)
  Memory6/1 -> Cruise/3(PCC_FGC_Te_0)
  Memory3/1 -> Cruise/4(PCC_FGC_ig_0)
  Sum2/1 -> Cruise/5(PCC_FGC_s_0)
  Memory5/1 -> Cruise/6(PCC_FGC_lambda_L0)
  Memory7/1 -> Cruise/7(PCC_FGC_lambda_U0)
  Memory4/1 -> Follow/1(PCC_GC_v_0)
  km/h2m/s_4/1 -> Follow/2(PCC_GC_vd_0)
  Memory13/1 -> Follow/3(PCC_GC_Te_0)
  Memory9/1 -> Follow/4(PCC_GC_ig_0)
  Sum1/1 -> Follow/5(PCC_GC_s_0)
  [LeaderRelaPos] -> Follow/6(PCC_GC_delta_s)
  [LeaderRelaSpd] -> Follow/7(PCC_GC_delta_v)
  Memory11/1 -> Follow/8(PCC_GC_lambda_L0)
  Memory14/1 -> Follow/9(PCC_GC_lambda_U0)
  Follow/7(PCC_Follow_lambda_L) -> Scope3/1
  Follow/8(PCC_Follow_lambda_U) -> Scope3/2
  PCC_FGC_Ne_0(rpm)/1 -> [PCC_FGC_Ne_0]
  [PCC_FGC_Ne_0] -> Coast/1(PCC_HX_Ne_0)
  [Mode_out] -> Compare To Constant/1
  Compare To Constant/1 -> Cruise/Enable
  [Mode_out] -> Compare To Constant1/1
  Compare To Constant1/1 -> Follow/Enable
  Compare To Constant2/1 -> Coast/Enable
  [Mode_out] -> Compare To Constant2/1
  Compare To Constant3/1 -> Brake/Enable
  [Mode_out] -> Compare To Constant3/1
  Bus Selector/3 -> Rate Limiter1/1  "<Tb>"
  Multiport Switch/1 -> Bus Selector/1
  [Mode_out] -> Multiport Switch/1
  Bus Creator/1 -> Multiport Switch/2
  Bus Creator1/1 -> Multiport Switch/3
  Bus Creator2/1 -> Multiport Switch/4
  Bus Creator3/1 -> Multiport Switch/5
  Cruise/1(PCC_Cruise_ne) -> [PCC_Cruise_ne]
  Cruise/2(PCC_Cruise_Te) -> Scope/1, [PCC_Cruise_Te]
  Cruise/3(PCC_Cruise_Tb) -> [PCC_Cruise_Tb]
  Cruise/4(PCC_Cruise_i) -> Scope2/1, [PCC_Cruise_i]
  Cruise/5(PCC_Cruise_MPC_active) -> [PCC_Cruise_MPC_active]
  Cruise/6(PCC_Cruise_lambda_opt) -> [PCC_Cruise_lambda_opt]
  [PCC_Cruise_ne] -> Bus Creator/1  "ne"
  [PCC_Cruise_Te] -> Bus Creator/2  "Te"
  [PCC_Cruise_MPC_active] -> Bus Creator/5  "MPC_active"
  [PCC_Cruise_lambda_opt] -> Bus Creator/6  "lambda_opt"
  [PCC_Cruise_Tb] -> Bus Creator/3  "Tb"
  [PCC_Cruise_i] -> Bus Creator/4  "i"
  Follow/5(PCC_Follow_MPC_active) -> [PCC_Follow_MPC_active]
  Follow/6(PCC_Follow_lambda_opt) -> [PCC_Follow_lambda_opt]
  Follow/1(PCC_Follow_ne) -> [PCC_Follow_ne]
  Follow/2(PCC_Follow_Te) -> Scope1/1, [PCC_Follow_Te]
  Follow/3(PCC_Follow_Tb) -> [PCC_Follow_Tb]
  Follow/4(PCC_Follow_i) -> [PCC_Follow_i]
  [PCC_Follow_Te] -> Bus Creator1/2  "Te"
  [PCC_Follow_ne] -> Bus Creator1/1  "ne"
  [PCC_Follow_MPC_active] -> Bus Creator1/5  "MPC_active"
  [PCC_Follow_lambda_opt] -> Bus Creator1/6  "lambda_opt"
  [PCC_Follow_Tb] -> Bus Creator1/3  "Tb"
  [PCC_Follow_i] -> Bus Creator1/4  "i"
  Coast/5(PCC_Coast_MPCState) -> [PCC_Coast_MPC_active]
  Coast/6(PCC_Coast_LambdaOpt) -> [PCC_Coast_lambda_opt]
  Coast/4(PCC_Coast_IterNum) -> [PCC_Coast_i]
  Coast/3(PCC_Coast_Tb) -> [PCC_Coast_Tb]
  Coast/2(PCC_Coast_Te) -> [PCC_Coast_Te]
  Coast/1(PCC_FGC_Ne) -> [PCC_Coast_ne]
  [PCC_Coast_ne] -> Bus Creator2/1  "ne"
  [PCC_Coast_MPC_active] -> Bus Creator2/5  "MPC_active"
  [PCC_Coast_lambda_opt] -> Bus Creator2/6  "lambda_opt"
  [PCC_Coast_Te] -> Bus Creator2/2  "Te"
  [PCC_Coast_Tb] -> Bus Creator2/3  "Tb"
  [PCC_Coast_i] -> Bus Creator2/4  "i"
  [PCC_FGC_v_0] -> km/h2m/s_6/1
  Memory15/1 -> Brake/1(PCC_ZD_v_0)
  km/h2m/s_6/1 -> Memory15/1
  [PCC_FGC_Ne_0] -> Brake/2(PCC_ZD_Ne_0)
  [LeaderRelaSpd] -> Brake/3(PCC_ZD_delta_v)
  [LeaderRelaPos] -> Brake/4(PCC_ZD_delta_s)
  Brake/1(PCC_Brake_Ne) -> [PCC_Brake_ne]
  Brake/2(PCC_Brake_Te) -> [PCC_Brake_Te]
  Brake/3(PCC_Brake_Tb) -> [PCC_Brake_Tb]
  Brake/5(PCC_Brake_MPCState) -> [PCC_Brake_MPC_active]
  Brake/6(PCC_Brake_LambdaOpt) -> [PCC_Brake_lambda_opt]
  Brake/4(PCC_Brake_IterNum) -> [PCC_Brake_i]
  [PCC_Brake_MPC_active] -> Bus Creator3/5  "MPC_active"
  [PCC_Brake_lambda_opt] -> Bus Creator3/6  "lambda_opt"
  [PCC_Brake_ne] -> Bus Creator3/1  "ne"
  [PCC_Brake_Te] -> Bus Creator3/2  "Te"
  [PCC_Brake_Tb] -> Bus Creator3/3  "Tb"
  [PCC_Brake_i] -> Bus Creator3/4  "i"
  [Mode_out] -> Mode_out/1
  Rate Limiter1/1 -> PCC_FGC_Tb/1
  [PCC_Cruise_lambda_opt] -> Memory5/1
  [PCC_Cruise_lambda_opt] -> Memory7/1
  [PCC_Follow_lambda_opt] -> Memory11/1
  [PCC_Follow_lambda_opt] -> Memory14/1

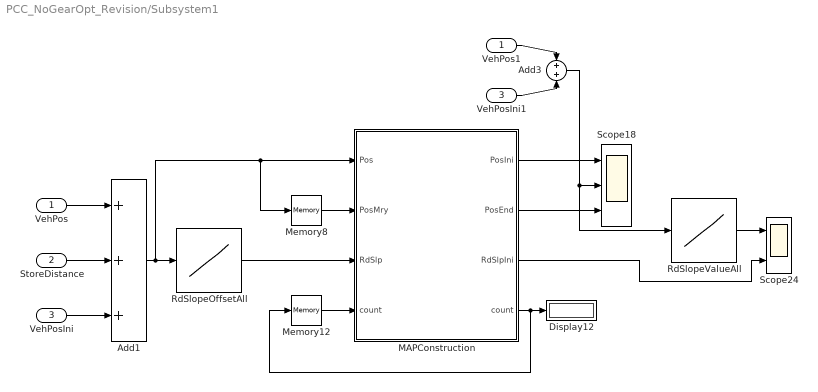
== system PCC_NoGearOpt_Revision/Subsystem1 ==
  VehPos : Inport
  StoreDistance : Inport  Port=2
  VehPosIni : Inport  Port=3
  Add1 : Sum  Inputs=+++
  Add3 : Sum
  Display12 : Display
  MAPConstruction : MATLAB Function  TreatAsAtomicUnit=on
  Memory12 : Memory
  Memory8 : Memory
  RdSlopeOffsetAll : Lookup_n-D  NumberOfTableDimensions=1  BreakpointsForDimension1=ParaMAP_RdSlopeOffsetAll  Table=ParaMAP_RdSlopeValueAll  InterpMethod=Nearest  InternalRulePriority=Speed  RndMeth=Simplest  InputSameDT=on
  RdSlopeValueAll : Lookup_n-D  NumberOfTableDimensions=1  BreakpointsForDimension1=ParaMAP_RdSlopeOffsetAll  Table=ParaMAP_RdSlopeValueAll  InterpMethod=Nearest  InternalRulePriority=Speed  RndMeth=Simplest  InputSameDT=on
  Scope18 : Scope  NumInputPorts=3
  Scope24 : Scope  NumInputPorts=2
  VehPos1 : InportShadow
  VehPosIni1 : InportShadow  Port=3
  wires:
  MAPConstruction/3(RdSlpIni) -> Scope24/2
  MAPConstruction/4(count) -> Memory12/1, Display12/1
  Memory8/1 -> MAPConstruction/2(PosMry)
  VehPos1/1 -> Add3/1
  Add3/1 -> RdSlopeValueAll/1, Scope18/2
  VehPosIni/1 -> Add1/3
  MAPConstruction/2(PosEnd) -> Scope18/3
  MAPConstruction/1(PosIni) -> Scope18/1
  Memory12/1 -> MAPConstruction/4("count ")
  Add1/1 -> RdSlopeOffsetAll/1, Memory8/1, MAPConstruction/1(Pos)
  VehPosIni1/1 -> Add3/2
  RdSlopeValueAll/1 -> Scope24/1
  StoreDistance/1 -> Add1/2
  VehPos/1 -> Add1/1
  RdSlopeOffsetAll/1 -> MAPConstruction/3(RdSlp)

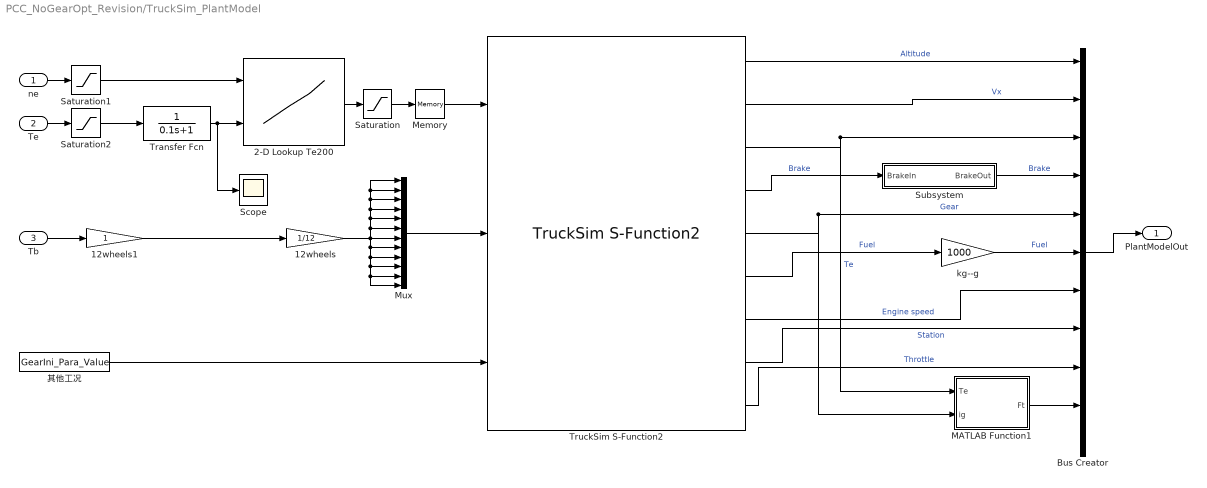
== system PCC_NoGearOpt_Revision/TruckSim_PlantModel ==
  ne : Inport
  Te : Inport  Port=2
  Tb : Inport  Port=3
  12wheels : Gain  Gain=1/12
  12wheels1 : Gain
  2-D Lookup Te200 : Lookup_n-D  BreakpointsForDimension1=[600,700,800,900,1000,1100,1200,1300,1400,1500,1600,1700,1800,1900,2000]  BreakpointsForDimension2=-400:50:2650  Table=[-0.0100000000000000,-0.00666666666666667,-0.00333333333333333,0,0.00333333333333333,0.00666666666666667,0.0100000000000000,0.0133333333333333,0.0166666666666667,0.0200000000000000,0.0266445182724252,0.0332890365448505,0.0399335548172758,0.0465780730897010,0.0532225913621262,0.0598671096345515,0.0665116279069768,0.0731561461794020,0.0798006644518273,0.0864451827242525,0.0930897009966777,0.0997342192691030,0.114035087719298,0.128654970760234,0.143274853801170,0.157894736842105,0.172514619883041,0.187134502923977,1,3.50000000000000,6,8.50000000000000,11,13.5000000000000,16,18.5000000000000,21,23.5000000000000,26,28.5000000000000,31,33.5000000000000,36,38.5000000000000,41,43.5000000000000,46,48.5000000000000,51,53.5000000000000,56,58.5000000000000,61,63.5000000000000,66,68.5000000000000,71,73.5000000000000,76,78.5000000000000,81,83.5000000000000;-0.00666666666666667,-0.00333333333333333,0,0.00333333333333333,0.00666666666666667,0.0100000000000000,0.0133333333333333,0.0166666666666667,0.0200000000000000,0.0272463768115942,0.0344927536231884,0.0417391304347826,0.0489855072463768,0.0562318840579710,0.0634782608695652,0.0707246376811594,0.0779710144927536,0.0852173913043478,0.0924637681159420,0.0997101449275362,0.111940298507463,0.124378109452736,0.136815920398010,0.149253731343284,0.161691542288557,0.174129353233831,0.186567164179105,0.199004975124378,0.212957746478873,0.227042253521127,0.241126760563380,0.255211267605634,0.269295774647887,0.283380281690141,0.297464788732394,0.311549295774648,0.325633802816901,0.339718309859155,0.353802816901408,0.367887323943662,0.381971830985916,0.396056338028169,2.50000000000000,5,7.50000000000000,10,12.5000000000000,15,17.5000000000000,20,22.5000000000000,25,27.5000000000000,30,32.5000000000000,35,37.5000000000000,40,42.5000000000000,45,47.5000000000000,50;-0.00333333333333333,0,0.00333333333333333,0.00666666666666667,0.0100000000000000,0.0133333333333333,0.0166666666666667,0.0200000000000000,0.0279681274900398,0.0359362549800797,0.0439043824701195,0.0518725099601594,0.0598406374501992,0.0678087649402391,0.0757768924302789,0.0837450199203187,0.0917131474103586,0.0996812749003984,0.111940298507463,0.124378109452736,0.136815920398010,0.149253731343284,0.161691542288557,0.174129353233831,0.186567164179105,0.199004975124378,0.211442786069652,0.223880597014925,0.236318407960199,0.248756218905473,0.261194029850746,0.273631840796020,0.286069651741294,0.298507462686567,0.310945273631841,0.323383084577114,0.335820895522388,0.348258706467662,0.360696517412935,0.373134328358209,0.385572139303483,0.398009950248756,0.412209302325581,0.426744186046512,0.441279069767442,0.455813953488372,0.470348837209302,0.484883720930233,0.499418604651163,0.972527472527473,1,1.02747252747253,1.05494505494506,1.08241758241758,1.10989010989011,1.13736263736264,1.16483516483517,1.19230769230769,1.21978021978022,1.24725274725275,1.27472527472527,1.30219780219780;0,0.00333333333333333,0.00666666666666667,0.0100000000000000,0.0133333333333333,0.0166666666666667,0.0200000000000000,0.0288495575221239,0.0376991150442478,0.0465486725663717,0.0553982300884956,0.0642477876106195,0.0730973451327434,0.0819469026548673,0.0907964601769912,0.0996460176991151,0.111940298507463,0.124378109452736,0.136815920398010,0.149253731343284,0.161691542288557,0.174129353233831,0.186567164179105,0.199004975124378,0.211442786069652,0.223880597014925,0.236318407960199,0.248756218905473,0.261194029850746,0.273631840796020,0.286069651741294,0.298507462686567,0.310945273631841,0.323383084577114,0.335820895522388,0.348258706467662,0.360696517412935,0.373134328358209,0.385572139303483,0.398009950248756,0.412209302325581,0.426744186046512,0.441279069767442,0.455813953488372,0.470348837209302,0.484883720930233,0.499418604651163,0.516438356164384,0.533561643835616,0.550684931506849,0.567808219178082,0.584931506849315,0.602061855670103,0.619243986254296,0.636426116838488,0.653608247422680,0.670790378006873,0.687972508591065,1,3.50000000000000,6,8.50000000000000;0 ...(+11561 chars)]  InternalRulePriority=Speed  RndMeth=Simplest  InputSameDT=on
  Bus Creator : BusCreator  Inputs=11
  MATLAB Function1 : MATLAB Function  TreatAsAtomicUnit=on
  Memory : Memory
  Mux : Mux  Inputs=12
  Saturation : Saturate  UpperLimit=1  LowerLimit=0
  Saturation1 : Saturate  UpperLimit=2000  LowerLimit=650
  Saturation2 : Saturate  UpperLimit=2650  LowerLimit=-400
  Scope : Scope
  Subsystem : Subsystem
  Transfer Fcn : TransferFcn  Denominator=[0.1 1]
  TruckSim S-Function2 : Solver_SF/TruckSim S-Function2  Priority=1  VehicleCode=s_ss__sss  SIMFILE=simfile.sim
      settings: AttributesFormatString=Vehicle Code: %<VehicleCode>
  kg--g : Gain  Gain=1000
  其他工况 : Constant  Value=GearIni_Para_Value
  PlantModelOut : Outport  VectorParamsAs1DForOutWhenUnconnected=off
  wires:
  12wheels/1 -> Mux/12, Mux/11, Mux/10, Mux/9, Mux/8, Mux/3, Mux/1, Mux/2, Mux/4, Mux/5, Mux/6, Mux/7
  其他工况/1 -> TruckSim S-Function2/3
  TruckSim S-Function2/7 -> Bus Creator/7  "Engine speed"
  TruckSim S-Function2/2 -> Bus Creator/2  "Vx"
  TruckSim S-Function2/4 -> Subsystem/1(BrakeIn)  "Brake"
  TruckSim S-Function2/6 -> kg--g/1  "Fuel"
  Mux/1 -> TruckSim S-Function2/2
  TruckSim S-Function2/1 -> Bus Creator/1  "Altitude"
  Saturation/1 -> Memory/1
  TruckSim S-Function2/8 -> Bus Creator/8  "Station"
  Subsystem/1(BrakeOut) -> Bus Creator/4  "Brake"
  2-D Lookup Te200/1 -> Saturation/1
  Tb/1 -> 12wheels1/1
  kg--g/1 -> Bus Creator/6  "Fuel"
  TruckSim S-Function2/9 -> Bus Creator/9  "Throttle"
  Bus Creator/1 -> PlantModelOut/1
  ne/1 -> Saturation1/1
  Te/1 -> Saturation2/1
  Memory/1 -> TruckSim S-Function2/1
  Transfer Fcn/1 -> Scope/1, 2-D Lookup Te200/2
  Saturation2/1 -> Transfer Fcn/1
  Saturation1/1 -> 2-D Lookup Te200/1
  MATLAB Function1/1(Ft) -> Bus Creator/10
  TruckSim S-Function2/3 -> MATLAB Function1/1(Te), Bus Creator/3  "Te"
  TruckSim S-Function2/5 -> Bus Creator/5, MATLAB Function1/2(ig)  "Gear"
  ? -> Bus Creator/11  "Qfuel"
  12wheels1/1 -> 12wheels/1

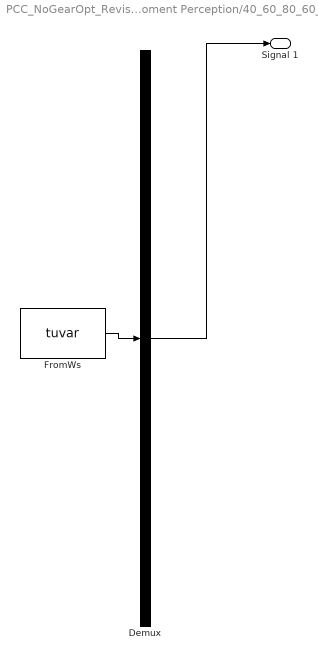
== system PCC_NoGearOpt_Revision/Enviroment Perception/40_60_80_60_40 ==
  Demux : Demux  Tag=STV Demux  Outputs=1
      settings: DisplayOption=none
  FromWs : FromWorkspace  Tag=STV FromWs  VariableName=tuvar
      SigBuilderData=|
      | common.afterFinalStr = 'Extrapolate'
      | common.sampleTime = 0
      | dataSet.timeRange = [0 2000]
      | dataSet.name = 'Group 1'
      | sbobj.Groups.Name = 'Group 1'
      | sbobj.Groups.Signals.Name = 'Signal 1'
      | sbobj.Groups.Signals.XData = [0 400 400 1200 1600 2000]
      | sbobj.Groups.Signals.YData = [60 60 80 80 80 80]
      | sbobj.Groups.TimeRange = [0 2000]
  Signal 1 : Outport  Tag=STV Outport
  wires:
  Demux/1 -> Signal 1/1
  FromWs/1 -> Demux/1

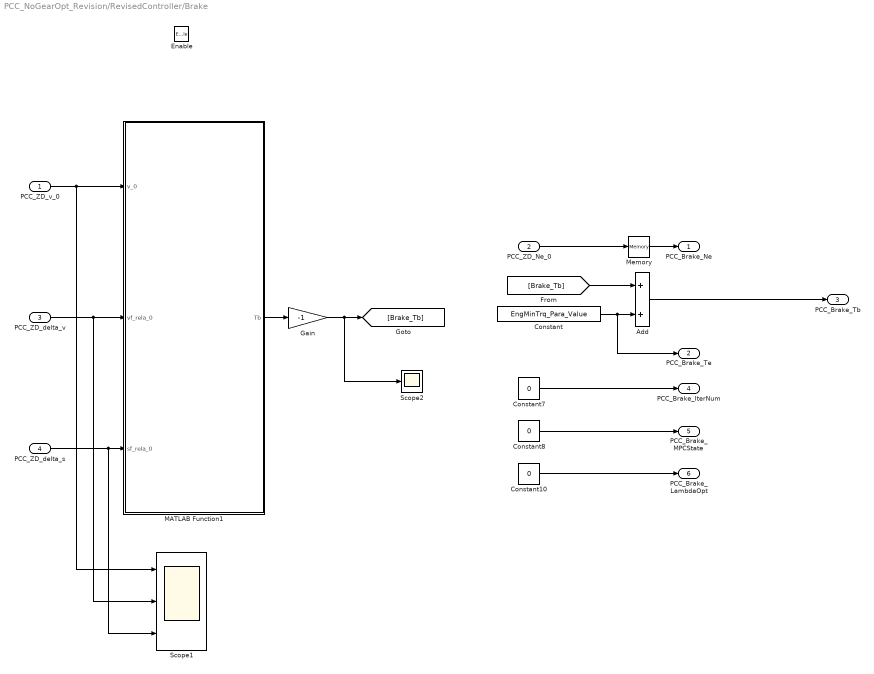
== system PCC_NoGearOpt_Revision/RevisedController/Brake ==
  PCC_ZD_v_0 : Inport
  PCC_ZD_Ne_0 : Inport  Port=2
  PCC_ZD_delta_v : Inport  Port=3
  PCC_ZD_delta_s : Inport  Port=4
  Enable : EnablePort
  Add : Sum
  Constant : Constant  Value=EngMinTrq_Para_Value
  Constant10 : Constant  Value=0
  Constant7 : Constant  Value=0
  Constant8 : Constant  Value=0
  Gain : Gain  Gain=-1
  MATLAB Function1 : MATLAB Function  TreatAsAtomicUnit=on
  Memory : Memory
  Scope1 : Scope  NumInputPorts=3
  Scope2 : Scope
  PCC_Brake_Ne : Outport
  PCC_Brake_Te : Outport  Port=2
  PCC_Brake_Tb : Outport  Port=3
  PCC_Brake_IterNum : Outport  Port=4
  PCC_Brake_MPCState : Outport  Port=5
  PCC_Brake_LambdaOpt : Outport  Port=6
  wires:
  MATLAB Function1/1(Tb) -> Gain/1
  Constant8/1 -> PCC_Brake_MPCState/1
  Constant10/1 -> PCC_Brake_LambdaOpt/1
  Constant7/1 -> PCC_Brake_IterNum/1
  PCC_ZD_delta_v/1 -> Scope1/2, MATLAB Function1/2(vf_rela_0)
  PCC_ZD_delta_s/1 -> Scope1/3, MATLAB Function1/3(sf_rela_0)
  PCC_ZD_v_0/1 -> MATLAB Function1/1(v_0), Scope1/1
  Memory/1 -> PCC_Brake_Ne/1
  PCC_ZD_Ne_0/1 -> Memory/1
  Gain/1 -> Scope2/1, [Brake_Tb]
  [Brake_Tb] -> Add/1
  Constant/1 -> PCC_Brake_Te/1, Add/2
  Add/1 -> PCC_Brake_Tb/1

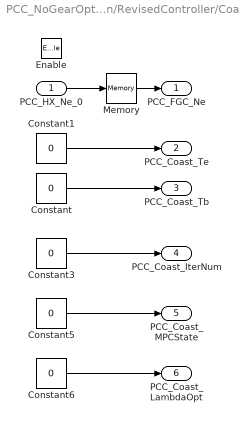
== system PCC_NoGearOpt_Revision/RevisedController/Coast ==
  PCC_HX_Ne_0 : Inport
  Enable : EnablePort
  Constant{,1,3,5..6} (5 alike) : Constant  Value=0
  Memory : Memory
  PCC_FGC_Ne : Outport
  PCC_Coast_Te : Outport  Port=2
  PCC_Coast_Tb : Outport  Port=3
  PCC_Coast_IterNum : Outport  Port=4
  PCC_Coast_MPCState : Outport  Port=5
  PCC_Coast_LambdaOpt : Outport  Port=6
  wires:
  Constant/1 -> PCC_Coast_Tb/1
  PCC_HX_Ne_0/1 -> Memory/1
  Constant3/1 -> PCC_Coast_IterNum/1
  Constant5/1 -> PCC_Coast_MPCState/1
  Constant6/1 -> PCC_Coast_LambdaOpt/1
  Memory/1 -> PCC_FGC_Ne/1
  Constant1/1 -> PCC_Coast_Te/1

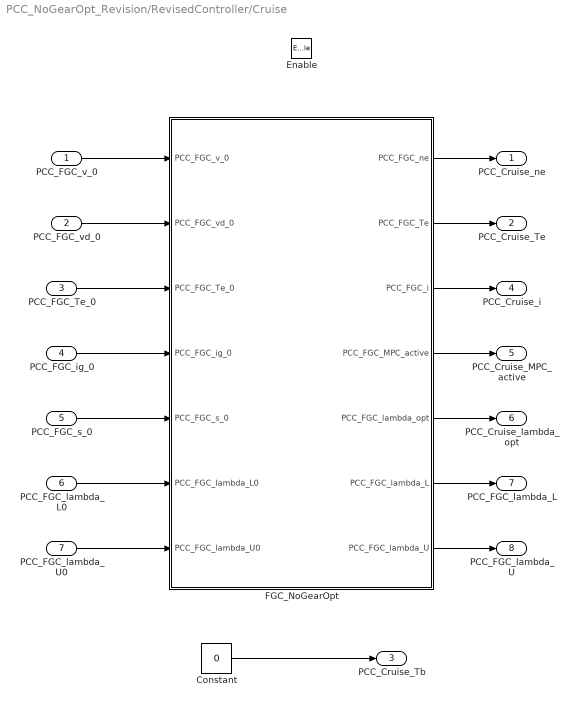
== system PCC_NoGearOpt_Revision/RevisedController/Cruise ==
  PCC_FGC_v_0 : Inport
  PCC_FGC_vd_0 : Inport  Port=2
  PCC_FGC_Te_0 : Inport  Port=3
  PCC_FGC_ig_0 : Inport  Port=4
  PCC_FGC_s_0 : Inport  Port=5
  PCC_FGC_lambda_L0 : Inport  Port=6
  PCC_FGC_lambda_U0 : Inport  Port=7
  Enable : EnablePort
  Constant : Constant  Value=0
  FGC_NoGearOpt : MATLAB Function  TreatAsAtomicUnit=on
  PCC_Cruise_ne : Outport
  PCC_Cruise_Te : Outport  Port=2
  PCC_Cruise_Tb : Outport  Port=3
  PCC_Cruise_i : Outport  Port=4
  PCC_Cruise_MPC_active : Outport  Port=5
  PCC_Cruise_lambda_opt : Outport  Port=6
  PCC_FGC_lambda_L : Outport  Port=7
  PCC_FGC_lambda_U : Outport  Port=8
  wires:
  PCC_FGC_s_0/1 -> FGC_NoGearOpt/5(PCC_FGC_s_0)
  FGC_NoGearOpt/1(PCC_FGC_ne) -> PCC_Cruise_ne/1
  PCC_FGC_lambda_L0/1 -> FGC_NoGearOpt/6(PCC_FGC_lambda_L0)
  FGC_NoGearOpt/3(PCC_FGC_i) -> PCC_Cruise_i/1
  FGC_NoGearOpt/5(PCC_FGC_lambda_opt) -> PCC_Cruise_lambda_opt/1
  FGC_NoGearOpt/4(PCC_FGC_MPC_active) -> PCC_Cruise_MPC_active/1
  FGC_NoGearOpt/2(PCC_FGC_Te) -> PCC_Cruise_Te/1
  PCC_FGC_Te_0/1 -> FGC_NoGearOpt/3(PCC_FGC_Te_0)
  PCC_FGC_vd_0/1 -> FGC_NoGearOpt/2(PCC_FGC_vd_0)
  FGC_NoGearOpt/7(PCC_FGC_lambda_U) -> PCC_FGC_lambda_U/1
  PCC_FGC_lambda_U0/1 -> FGC_NoGearOpt/7(PCC_FGC_lambda_U0)
  PCC_FGC_v_0/1 -> FGC_NoGearOpt/1(PCC_FGC_v_0)
  PCC_FGC_ig_0/1 -> FGC_NoGearOpt/4(PCC_FGC_ig_0)
  FGC_NoGearOpt/6(PCC_FGC_lambda_L) -> PCC_FGC_lambda_L/1
  Constant/1 -> PCC_Cruise_Tb/1
